simulink library "ann"  (Simulink 3.00)
undefined symbols (not defined in the file): V0, W0
libraries: simulink3 x3, neural x1
(part 2 of 2)

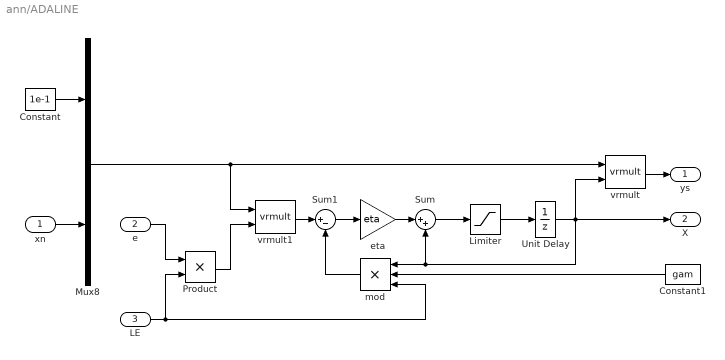
== system ann/ADALINE ==
  xn : Inport  Port=1  PortWidth=-1  SampleTime=-1  DataType=auto
      settings: SignalType=auto
  e : Inport  Port=2  PortWidth=-1  SampleTime=-1  DataType=auto
      settings: SignalType=auto
  LE : Inport  Port=3  PortWidth=-1  SampleTime=-1  DataType=auto
      settings: SignalType=auto
  Constant : Constant  Value=1e-1
  Constant1 : Constant  Orientation=left  Value=gam
  Limiter : Saturate  UpperLimit=L  LowerLimit=-L
  Mux8 : Mux  Inputs=2
  Product : Product  Inputs=2  SaturateOnIntegerOverflow=on
  Sum : Sum  Inputs=|++  SaturateOnIntegerOverflow=on
  Sum1 : Sum  Inputs=|+-  SaturateOnIntegerOverflow=on
  Unit Delay : UnitDelay  X0=W(:)  SampleTime=T
  eta : Gain  Gain=eta  SaturateOnIntegerOverflow=on
  mod : Product  Orientation=left  Inputs=3  SaturateOnIntegerOverflow=on
  vrmult : S-Function  FunctionName=vrmult  Parameters=dims  PortCounts=[]  SFunctionModules=''  mask(Simulink Matrix Library Block){dims=[1 ni+1 no]}
      mask prompts: dims "[n p m]"
      mask help:
      | Real Varying Matrices Multiplication
      |   Input 1   : elements of matrix X (n by p)
      |   Input 2   : elements of matrix Y (p by m)
      |   Output   : elements of matrix X*Y (n by m)
      mask Help:
      | <p>
      | Elements of input and output matrices are taken columnwise.
      | </p>
      | <p>
      | To use this block you should have the smxl library in your path.
      | </p>
      mask Display: disp('Z=X*Y')
  vrmult1 : S-Function  FunctionName=vrmult  Parameters=dims  PortCounts=[]  SFunctionModules=''  mask(Simulink Matrix Library Block){dims=[ni+1 1 no]}
      mask prompts: dims "[n p m]"
      mask help:
      | Real Varying Matrices Multiplication
      |   Input 1   : elements of matrix X (n by p)
      |   Input 2   : elements of matrix Y (p by m)
      |   Output   : elements of matrix X*Y (n by m)
      mask Help:
      | <p>
      | Elements of input and output matrices are taken columnwise.
      | </p>
      | <p>
      | To use this block you should have the smxl library in your path.
      | </p>
      mask Display: disp('Z=X*Y')
  ys : Outport  Port=1
  X : Outport  Port=2
  wires:
  Limiter/1 -> Unit Delay/1
  Sum/1 -> Limiter/1
  Unit Delay/1 -> vrmult/2, Sum/2, mod/1, X/1
  vrmult/1 -> ys/1
  Constant1/1 -> mod/2
  eta/1 -> Sum/1
  Sum1/1 -> eta/1
  vrmult1/1 -> Sum1/1
  mod/1 -> Sum1/2
  Product/1 -> vrmult1/2
  e/1 -> Product/1
  LE/1 -> Product/2, mod/3
  Mux8/1 -> vrmult/1, vrmult1/1
  xn/1 -> Mux8/2
  Constant/1 -> Mux8/1

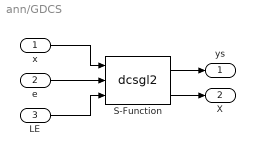
== system ann/GDCS ==
  x : Inport  Port=1  PortWidth=-1  SampleTime=-1  DataType=auto
      settings: SignalType=auto
  e : Inport  Port=2  PortWidth=-1  SampleTime=-1  DataType=auto
      settings: SignalType=auto
  LE : Inport  Port=3  PortWidth=-1  SampleTime=-1  DataType=auto
      settings: SignalType=auto
  S-Function : S-Function  FunctionName=dcsgl2  Parameters=Dim,norlat,eta,lim,real(lga),S,T  PortCounts=[]  SFunctionModules=''
  ys : Outport  Port=1
  X : Outport  Port=2
  wires:
  S-Function/1 -> ys/1
  S-Function/2 -> X/1
  x/1 -> S-Function/1
  e/1 -> S-Function/2
  LE/1 -> S-Function/3

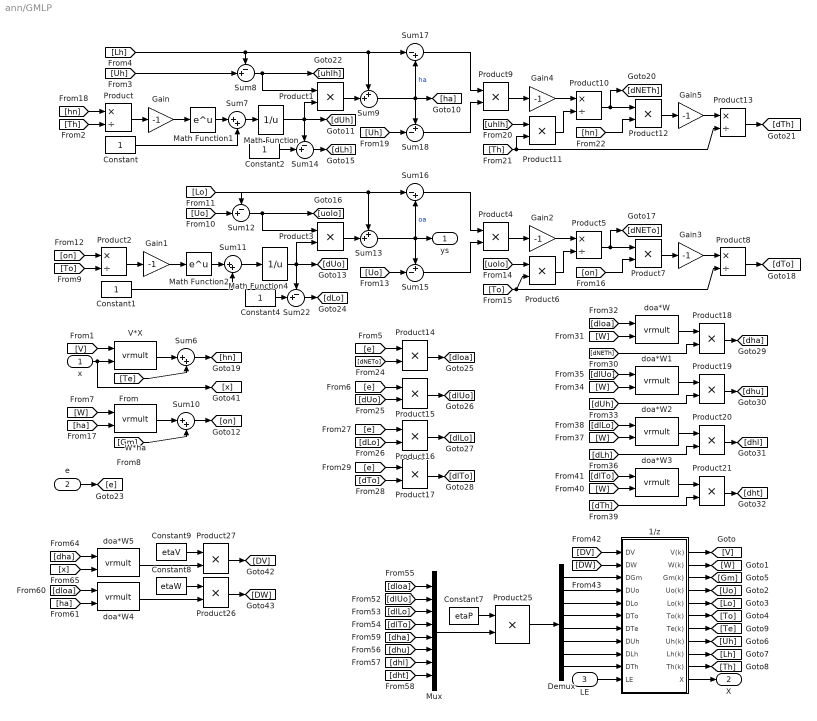
== system ann/GMLP ==
  x : Inport  Port=1  PortWidth=-1  SampleTime=-1  DataType=auto
      settings: SignalType=auto
  e : Inport  Port=2  PortWidth=-1  SampleTime=-1  DataType=auto
      settings: SignalType=auto
  LE : Inport  Port=3  PortWidth=-1  SampleTime=-1  DataType=auto
      settings: SignalType=auto
  1/z : Subsystem
  Constant{,1..2,4} (4 alike) : Constant  Value=1
  Constant7 : Constant  Value=etaP
  Constant8 : Constant  Value=etaW
  Constant9 : Constant  Value=etaV
  Demux : Demux  Outputs=8
  Gain{,1..5} (6 alike) : Gain  Gain=-1  SaturateOnIntegerOverflow=on
  Math Function : Math  Operator=reciprocal  OutputSignalType=auto
  Math Function1 : Math  Operator=exp  OutputSignalType=auto
  Math Function2 : Math  Operator=exp  OutputSignalType=auto
  Math Function4 : Math  Operator=reciprocal  OutputSignalType=auto
  Mux : Mux  Inputs=8
  Product{,2,5,8,10,13} (6 alike) : Product  Inputs=*/  SaturateOnIntegerOverflow=on
  Product{1,3..4,6..7,9,11..12,14..21,25..27} (19 alike) : Product  Inputs=**  SaturateOnIntegerOverflow=on
  Sum{6..7,10..11} (4 alike) : Sum  Inputs=|++  SaturateOnIntegerOverflow=on
  Sum{8,12,14,22} (4 alike) : Sum  Inputs=-+|  SaturateOnIntegerOverflow=on
  Sum13 : Sum  Inputs=++|  SaturateOnIntegerOverflow=on
  Sum15 : Sum  Inputs=+-|  SaturateOnIntegerOverflow=on
  Sum16 : Sum  Inputs=|-+  SaturateOnIntegerOverflow=on
  Sum17 : Sum  Inputs=|-+  SaturateOnIntegerOverflow=on
  Sum18 : Sum  Inputs=+-|  SaturateOnIntegerOverflow=on
  Sum9 : Sum  Inputs=++|  SaturateOnIntegerOverflow=on
  V*X : S-Function  FunctionName=vrmult  Parameters=dims  PortCounts=[]  SFunctionModules=''  mask(Simulink Matrix Library Block){dims=[nh ni 1]}
      mask prompts: dims "[n p m]"
      mask help:
      | Real Varying Matrices Multiplication
      |   Input 1   : elements of matrix X (n by p)
      |   Input 2   : elements of matrix Y (p by m)
      |   Output   : elements of matrix X*Y (n by m)
      mask Help:
      | <p>
      | Elements of input and output matrices are taken columnwise.
      | </p>
      | <p>
      | To use this block you should have the smxl library in your path.
      | </p>
      mask Display: disp('Z=X*Y')
  W*ha : S-Function  FunctionName=vrmult  Parameters=dims  PortCounts=[]  SFunctionModules=''  mask(Simulink Matrix Library Block){dims=[no nh 1]}
      mask prompts: dims "[n p m]"
      mask help:
      | Real Varying Matrices Multiplication
      |   Input 1   : elements of matrix X (n by p)
      |   Input 2   : elements of matrix Y (p by m)
      |   Output   : elements of matrix X*Y (n by m)
      mask Help:
      | <p>
      | Elements of input and output matrices are taken columnwise.
      | </p>
      | <p>
      | To use this block you should have the smxl library in your path.
      | </p>
      mask Display: disp('Z=X*Y')
  doa*W : S-Function  FunctionName=vrmult  Parameters=dims  PortCounts=[]  SFunctionModules=''  mask(Simulink Matrix Library Block){dims=[1 no nh]}
      mask prompts: dims "[n p m]"
      mask help:
      | Real Varying Matrices Multiplication
      |   Input 1   : elements of matrix X (n by p)
      |   Input 2   : elements of matrix Y (p by m)
      |   Output   : elements of matrix X*Y (n by m)
      mask Help:
      | <p>
      | Elements of input and output matrices are taken columnwise.
      | </p>
      | <p>
      | To use this block you should have the smxl library in your path.
      | </p>
      mask Display: disp('Z=X*Y')
  doa*W1 : S-Function  FunctionName=vrmult  Parameters=dims  PortCounts=[]  SFunctionModules=''  mask(Simulink Matrix Library Block){dims=[1 no nh]}
      mask prompts: dims "[n p m]"
      mask help:
      | Real Varying Matrices Multiplication
      |   Input 1   : elements of matrix X (n by p)
      |   Input 2   : elements of matrix Y (p by m)
      |   Output   : elements of matrix X*Y (n by m)
      mask Help:
      | <p>
      | Elements of input and output matrices are taken columnwise.
      | </p>
      | <p>
      | To use this block you should have the smxl library in your path.
      | </p>
      mask Display: disp('Z=X*Y')
  doa*W2 : S-Function  FunctionName=vrmult  Parameters=dims  PortCounts=[]  SFunctionModules=''  mask(Simulink Matrix Library Block){dims=[1 no nh]}
      mask prompts: dims "[n p m]"
      mask help:
      | Real Varying Matrices Multiplication
      |   Input 1   : elements of matrix X (n by p)
      |   Input 2   : elements of matrix Y (p by m)
      |   Output   : elements of matrix X*Y (n by m)
      mask Help:
      | <p>
      | Elements of input and output matrices are taken columnwise.
      | </p>
      | <p>
      | To use this block you should have the smxl library in your path.
      | </p>
      mask Display: disp('Z=X*Y')
  doa*W3 : S-Function  FunctionName=vrmult  Parameters=dims  PortCounts=[]  SFunctionModules=''  mask(Simulink Matrix Library Block){dims=[1 no nh]}
      mask prompts: dims "[n p m]"
      mask help:
      | Real Varying Matrices Multiplication
      |   Input 1   : elements of matrix X (n by p)
      |   Input 2   : elements of matrix Y (p by m)
      |   Output   : elements of matrix X*Y (n by m)
      mask Help:
      | <p>
      | Elements of input and output matrices are taken columnwise.
      | </p>
      | <p>
      | To use this block you should have the smxl library in your path.
      | </p>
      mask Display: disp('Z=X*Y')
  doa*W4 : S-Function  FunctionName=vrmult  Parameters=dims  PortCounts=[]  SFunctionModules=''  mask(Simulink Matrix Library Block){dims=[no 1 nh]}
      mask prompts: dims "[n p m]"
      mask help:
      | Real Varying Matrices Multiplication
      |   Input 1   : elements of matrix X (n by p)
      |   Input 2   : elements of matrix Y (p by m)
      |   Output   : elements of matrix X*Y (n by m)
      mask Help:
      | <p>
      | Elements of input and output matrices are taken columnwise.
      | </p>
      | <p>
      | To use this block you should have the smxl library in your path.
      | </p>
      mask Display: disp('Z=X*Y')
  doa*W5 : S-Function  FunctionName=vrmult  Parameters=dims  PortCounts=[]  SFunctionModules=''  mask(Simulink Matrix Library Block){dims=[nh 1 ni]}
      mask prompts: dims "[n p m]"
      mask help:
      | Real Varying Matrices Multiplication
      |   Input 1   : elements of matrix X (n by p)
      |   Input 2   : elements of matrix Y (p by m)
      |   Output   : elements of matrix X*Y (n by m)
      mask Help:
      | <p>
      | Elements of input and output matrices are taken columnwise.
      | </p>
      | <p>
      | To use this block you should have the smxl library in your path.
      | </p>
      mask Display: disp('Z=X*Y')
  ys : Outport  Port=1
  X : Outport  Port=2
  wires:
  Sum10/1 -> [on]
  1/z/11(X) -> X/1
  Product25/1 -> Demux/1
  Math Function2/1 -> Sum11/1
  Gain1/1 -> Math Function2/1
  1/z/10(Th(k)) -> [Th]
  1/z/9(Lh(k)) -> [Lh]
  1/z/8(Uh(k)) -> [Uh]
  1/z/7(Te(k)) -> [Te]
  1/z/6(To(k)) -> [To]
  1/z/5(Lo(k)) -> [Lo]
  1/z/4(Uo(k)) -> [Uo]
  1/z/3(Gm(k)) -> [Gm]
  1/z/2(W(k)) -> [W]
  1/z/1(V(k)) -> [V]
  [DV] -> 1/z/1(DV)
  [DW] -> 1/z/2(DW)
  Product27/1 -> [DV]
  Product26/1 -> [DW]
  doa*W4/1 -> Product26/2
  Constant8/1 -> Product26/1
  [dloa] -> doa*W4/1
  doa*W5/1 -> Product27/2
  Constant9/1 -> Product27/1
  [x] -> doa*W5/2
  [dha] -> doa*W5/1
  [ha] -> doa*W4/2
  Product18/1 -> [dha]
  Product17/1 -> [dlTo]
  [e] -> Product17/1
  Product16/1 -> [dlLo]
  [dLo] -> Product16/2
  [e] -> Product16/1
  Product15/1 -> [dlUo]
  [dUo] -> Product15/2
  [e] -> Product15/1
  Product14/1 -> [dloa]
  [dNETo] -> Product14/2
  [e] -> Product14/1
  x/1 -> [x], V*X/2
  Sum6/1 -> [hn]
  [V] -> V*X/1
  [Te] -> Sum6/2
  V*X/1 -> Sum6/1
  [ha] -> W*ha/2
  W*ha/1 -> Sum10/1
  [W] -> W*ha/1
  [Gm] -> Sum10/2
  [dTh] -> Product21/2
  Product21/1 -> [dht]
  doa*W3/1 -> Product21/1
  [W] -> doa*W3/2
  [dlTo] -> doa*W3/1
  [dLh] -> Product20/2
  Product20/1 -> [dhl]
  doa*W2/1 -> Product20/1
  [W] -> doa*W2/2
  [dlLo] -> doa*W2/1
  [dUh] -> Product19/2
  Product19/1 -> [dhu]
  doa*W1/1 -> Product19/1
  [W] -> doa*W1/2
  [dlUo] -> doa*W1/1
  [dNETh] -> Product18/2
  doa*W/1 -> Product18/1
  [W] -> doa*W/2
  [dloa] -> doa*W/1
  [dTo] -> Product17/2
  Sum22/1 -> [dLo]
  Constant4/1 -> Sum22/2
  Sum11/1 -> Math Function4/1
  [Lo] -> Sum16/1, Sum13/1, Sum12/1
  [Uo] -> Sum12/2
  Math Function4/1 -> Sum22/1, [dUo], Product3/2
  [on] -> Product2/1
  Constant1/1 -> Sum11/2
  Product2/1 -> Gain1/1
  [To] -> Product2/2
  Sum13/1 -> ys/1, Sum15/1, Sum16/2  "oa"
  Product3/1 -> Sum13/2
  [To] -> Product8/2, Product6/2
  Gain3/1 -> Product8/1
  Product7/1 -> Gain3/1
  Product5/1 -> Product7/1, [dNETo]
  Product6/1 -> Product5/2
  [uolo] -> Product6/1
  Gain2/1 -> Product5/1
  Sum12/1 -> [uolo], Product3/1
  Product4/1 -> Gain2/1
  Sum15/1 -> Product4/2
  Sum16/1 -> Product4/1
  [Uo] -> Sum15/2
  Product8/1 -> [dTo]
  Sum17/1 -> Product9/1
  Sum8/1 -> [uhlh], Product1/1
  [Lh] -> Sum17/1, Sum9/1, Sum8/1
  [Uh] -> Sum8/2
  Sum9/1 -> Sum18/1, [ha], Sum17/2  "ha"
  Product1/1 -> Sum9/2
  [Th] -> Product11/2, Product13/2
  Gain5/1 -> Product13/1
  Product12/1 -> Gain5/1
  [hn] -> Product12/2
  Product10/1 -> [dNETh], Product12/1
  Product11/1 -> Product10/2
  [uhlh] -> Product11/1
  Gain4/1 -> Product10/1
  Product9/1 -> Gain4/1
  Sum18/1 -> Product9/2
  Product13/1 -> [dTh]
  [Uh] -> Sum18/2
  [hn] -> Product/1
  Constant2/1 -> Sum14/2
  Sum14/1 -> [dLh]
  Math Function/1 -> Product1/2, Sum14/1, [dUh]
  Sum7/1 -> Math Function/1
  Constant/1 -> Sum7/2
  Math Function1/1 -> Sum7/1
  Gain/1 -> Math Function1/1
  Product/1 -> Gain/1
  [Th] -> Product/2
  Demux/1 -> 1/z/3(DGm)
  Demux/8 -> 1/z/10(DTh)
  Demux/7 -> 1/z/9(DLh)
  Demux/6 -> 1/z/8(DUh)
  Demux/5 -> 1/z/7(DTe)
  Demux/4 -> 1/z/6(DTo)
  Demux/3 -> 1/z/5(DLo)
  Demux/2 -> 1/z/4(DUo)
  e/1 -> [e]
  LE/1 -> 1/z/11(LE)
  Constant7/1 -> Product25/1
  [dht] -> Mux/8
  [dhl] -> Mux/7
  [dhu] -> Mux/6
  [dha] -> Mux/5
  [dlTo] -> Mux/4
  [dlLo] -> Mux/3
  [dloa] -> Mux/1
  [dlUo] -> Mux/2
  Mux/1 -> Product25/2
  [on] -> Product7/2

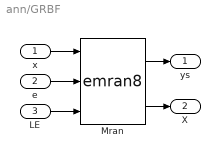
== system ann/GRBF ==
  x : Inport  Port=1  PortWidth=-1  SampleTime=-1  DataType=auto
      settings: SignalType=auto
  e : Inport  Port=2  PortWidth=-1  SampleTime=-1  DataType=auto
      settings: SignalType=auto
  LE : Inport  Port=3  PortWidth=-1  SampleTime=-1  DataType=auto
      settings: SignalType=auto
  Mran : S-Function  FunctionName=emran8  Parameters=real(dim(:)),real(nwrap(:)),real(eta(:)),real(gam(:)),real(lim(:)),real(e1(:)),real(e2(:)),real(e3(:)),real(x0(:)),real(T(:))  PortCounts=[]  SFunctionModules=''
  ys : Outport  Port=1
  X : Outport  Port=2
  wires:
  Mran/1 -> ys/1
  Mran/2 -> X/1
  x/1 -> Mran/1
  e/1 -> Mran/2
  LE/1 -> Mran/3

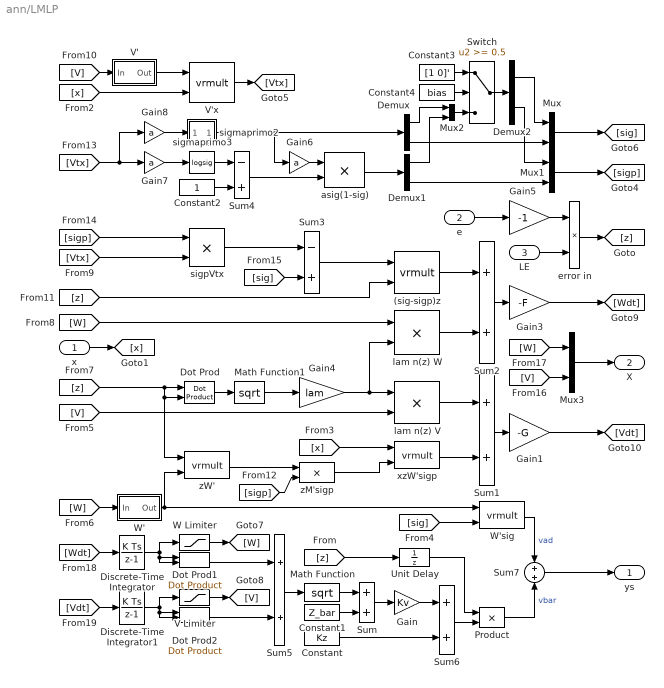
== system ann/LMLP ==
  x : Inport  Port=1  PortWidth=-1  SampleTime=-1  DataType=auto
      settings: SignalType=auto
  e : Inport  Port=2  PortWidth=-1  SampleTime=-1  DataType=auto
      settings: SignalType=auto
  LE : Inport  Port=3  PortWidth=-1  SampleTime=-1  DataType=auto
      settings: SignalType=auto
  (sig-sigp)z : S-Function  FunctionName=vrmult  Parameters=dims  PortCounts=[]  SFunctionModules=''  mask(Simulink Matrix Library Block){dims=[nnh 1 nno]}
      mask prompts: dims "[n p m]"
      mask help:
      | Real Varying Matrices Multiplication
      |   Input 1   : elements of matrix X (n by p)
      |   Input 2   : elements of matrix Y (p by m)
      |   Output   : elements of matrix X*Y (n by m)
      mask Help:
      | <p>
      | Elements of input and output matrices are taken columnwise.
      | </p>
      | <p>
      | To use this block you should have the smxl library in your path.
      | </p>
      mask Display: disp('Z=X*Y')
  Constant : Constant  Value=Kz
  Constant1 : Constant  Value=Z_bar
  Constant2 : Constant  Value=1
  Constant3 : Constant  Value=[1 0]'
  Constant4 : Constant  Value=bias
  Demux : Demux  Outputs=[1 nnh-1]
  Demux1 : Demux  Outputs=[1 nnh-1]
  Demux2 : Demux  Outputs=[1 1]
  Discrete-Time Integrator : DiscreteIntegrator  IntegratorMethod=ForwardEuler  ExternalReset=none  InitialConditionSource=internal  InitialCondition=W0(:)  LimitOutput=off  UpperSaturationLimit=inf  LowerSaturationLimit=-inf  ShowSaturationPort=off  ShowStatePort=off  SampleTime=T
  Discrete-Time Integrator1 : DiscreteIntegrator  IntegratorMethod=ForwardEuler  ExternalReset=none  InitialConditionSource=internal  InitialCondition=V0(:)  LimitOutput=off  UpperSaturationLimit=inf  LowerSaturationLimit=-inf  ShowSaturationPort=off  ShowStatePort=off  SampleTime=T
  Dot Prod : simulink3/Math/Dot Product
  Dot Prod1 : simulink3/Math/Dot Product
  Dot Prod2 : simulink3/Math/Dot Product
  Gain : Gain  Gain=Kv  SaturateOnIntegerOverflow=on
  Gain1 : Gain  Gain=-G  SaturateOnIntegerOverflow=on
  Gain3 : Gain  Gain=-F  SaturateOnIntegerOverflow=on
  Gain4 : Gain  Gain=lam  SaturateOnIntegerOverflow=on
  Gain5 : Gain  Gain=-1  SaturateOnIntegerOverflow=on
  Gain6 : Gain  Gain=a  SaturateOnIntegerOverflow=on
  Gain7 : Gain  Gain=a  SaturateOnIntegerOverflow=on
  Gain8 : Gain  Gain=a  SaturateOnIntegerOverflow=on
  Math Function : Math  Operator=sqrt  OutputSignalType=real
  Math Function1 : Math  Operator=sqrt  OutputSignalType=real
  Mux : Mux  Inputs=[1 nnh-1]
  Mux1 : Mux  Inputs=[1 nnh-1]
  Mux2 : Mux  Inputs=[1 1]
  Mux3 : Mux  Inputs=2
  Product : Product  Inputs=2  SaturateOnIntegerOverflow=on
  Sum{,1..2,5..6} (5 alike) : Sum  Inputs=++  SaturateOnIntegerOverflow=on
  Sum3 : Sum  Inputs=-+  SaturateOnIntegerOverflow=on
  Sum4 : Sum  Inputs=-+  SaturateOnIntegerOverflow=on
  Sum7 : Sum  Inputs=+|+  SaturateOnIntegerOverflow=on
  Switch : Switch  Threshold=0.5
  Unit Delay : UnitDelay  X0=0  SampleTime=T
  V Limiter : Saturate  UpperLimit=LV  LowerLimit=-LV
  V' : Subsystem  mask(Simulink Matrix Library Block){dims=[nni nnh]}
      mask prompts: dims "[n m]"
      mask help:
      | Real Varying Matrix Transposition
      |   Input      : elements of matrix X (n by m)
      |   Output   : elements of matrix X' (m by n)
      mask Help:
      | <p>
      | Elements of input and output matrices are taken columnwise.
      | </p>
      | <p>
      | To use this block you should have the smxl library in your path.
      | </p>
      mask Display: disp('Y=X''')
  V'x : S-Function  FunctionName=vrmult  Parameters=dims  PortCounts=[]  SFunctionModules=''  mask(Simulink Matrix Library Block){dims=[nnh nni 1]}
      mask prompts: dims "[n p m]"
      mask help:
      | Real Varying Matrices Multiplication
      |   Input 1   : elements of matrix X (n by p)
      |   Input 2   : elements of matrix Y (p by m)
      |   Output   : elements of matrix X*Y (n by m)
      mask Help:
      | <p>
      | Elements of input and output matrices are taken columnwise.
      | </p>
      | <p>
      | To use this block you should have the smxl library in your path.
      | </p>
      mask Display: disp('Z=X*Y')
  W Limiter : Saturate  UpperLimit=LW  LowerLimit=-LW
  W' : Subsystem  mask(Simulink Matrix Library Block){dims=[nnh nno]}
      mask prompts: dims "[n m]"
      mask help:
      | Real Varying Matrix Transposition
      |   Input      : elements of matrix X (n by m)
      |   Output   : elements of matrix X' (m by n)
      mask Help:
      | <p>
      | Elements of input and output matrices are taken columnwise.
      | </p>
      | <p>
      | To use this block you should have the smxl library in your path.
      | </p>
      mask Display: disp('Y=X''')
  W'sig : S-Function  FunctionName=vrmult  Parameters=dims  PortCounts=[]  SFunctionModules=''  mask(Simulink Matrix Library Block){dims=[nno nnh 1]}
      mask prompts: dims "[n p m]"
      mask help:
      | Real Varying Matrices Multiplication
      |   Input 1   : elements of matrix X (n by p)
      |   Input 2   : elements of matrix Y (p by m)
      |   Output   : elements of matrix X*Y (n by m)
      mask Help:
      | <p>
      | Elements of input and output matrices are taken columnwise.
      | </p>
      | <p>
      | To use this block you should have the smxl library in your path.
      | </p>
      mask Display: disp('Z=X*Y')
  asig(1-sig) : Product  Inputs=2  SaturateOnIntegerOverflow=on
  error in : Product  Inputs=2  SaturateOnIntegerOverflow=on
  lam n(z) V : Product  Inputs=2  SaturateOnIntegerOverflow=on
  lam n(z) W : Product  Inputs=2  SaturateOnIntegerOverflow=on
  sigmaprimo2 : Subsystem
      mask Description: Log sigmoid transfer function
      mask Display: plot([-1 1],[0 0],[-1 -.9 -.8 -.7 -.6 -.5 -.4 -.3 -.2 -.1 0 .1 .2 .3 .4 .5 .6 .7 .8 .9 1],1./(1+exp(-8*[-1 -.9 -.8 -.7 -.6 -.5 -.4 -.3 -.2 -.1 0 .1 .2 .3 .4 .5 .6 .7 .8 .9 1]))+.01)
  sigmaprimo3 : neural/Transfer Functions/logsig
  sigpVtx : Product  Inputs=2  SaturateOnIntegerOverflow=on
  xzW'sigp : S-Function  FunctionName=vrmult  Parameters=dims  PortCounts=[]  SFunctionModules=''  mask(Simulink Matrix Library Block){dims=[nni 1 nnh]}
      mask prompts: dims "[n p m]"
      mask help:
      | Real Varying Matrices Multiplication
      |   Input 1   : elements of matrix X (n by p)
      |   Input 2   : elements of matrix Y (p by m)
      |   Output   : elements of matrix X*Y (n by m)
      mask Help:
      | <p>
      | Elements of input and output matrices are taken columnwise.
      | </p>
      | <p>
      | To use this block you should have the smxl library in your path.
      | </p>
      mask Display: disp('Z=X*Y')
  zM'sigp : Product  Inputs=2  SaturateOnIntegerOverflow=on
  zW' : S-Function  FunctionName=vrmult  Parameters=dims  PortCounts=[]  SFunctionModules=''  mask(Simulink Matrix Library Block){dims=[1 nno nnh]}
      mask prompts: dims "[n p m]"
      mask help:
      | Real Varying Matrices Multiplication
      |   Input 1   : elements of matrix X (n by p)
      |   Input 2   : elements of matrix Y (p by m)
      |   Output   : elements of matrix X*Y (n by m)
      mask Help:
      | <p>
      | Elements of input and output matrices are taken columnwise.
      | </p>
      | <p>
      | To use this block you should have the smxl library in your path.
      | </p>
      mask Display: disp('Z=X*Y')
  ys : Outport  Port=1
  X : Outport  Port=2
  wires:
  Gain5/1 -> error in/1
  e/1 -> Gain5/1
  Unit Delay/1 -> Product/1
  [z] -> Unit Delay/1
  [V] -> lam n(z) V/2
  x/1 -> [x]
  [V] -> V'/1(In)
  V'/1(Out) -> V'x/1
  [x] -> V'x/2
  V'x/1 -> [Vtx]
  Constant3/1 -> Switch/1
  Constant4/1 -> Switch/2
  Mux2/1 -> Switch/3
  Switch/1 -> Demux2/1
  Demux2/2 -> Mux1/1
  Demux2/1 -> Mux/1
  Demux/1 -> Mux2/1
  Demux1/1 -> Mux2/2
  error in/1 -> [z]
  LE/1 -> error in/2
  [W] -> Mux3/1
  [V] -> Mux3/2
  Mux3/1 -> X/1
  Constant1/1 -> Sum/2
  Math Function/1 -> Sum/1
  Sum/1 -> Gain/1
  Gain/1 -> Sum6/1
  Constant/1 -> Sum6/2
  Sum6/1 -> Product/2
  [sig] -> W'sig/2
  W'sig/1 -> Sum7/1  "vad"
  Product/1 -> Sum7/2  "vbar"
  Sum5/1 -> Math Function/1
  V Limiter/1 -> [V]
  W Limiter/1 -> [W]
  [Vdt] -> Discrete-Time Integrator1/1
  [Wdt] -> Discrete-Time Integrator/1
  Dot Prod2/1 -> Sum5/2
  Dot Prod1/1 -> Sum5/1
  [W] -> W'/1(In)
  Sum7/1 -> ys/1
  Gain1/1 -> [Vdt]
  Sum2/1 -> Gain3/1
  (sig-sigp)z/1 -> Sum2/1
  lam n(z) W/1 -> Sum2/2
  Gain4/1 -> lam n(z) V/1, lam n(z) W/2
  [z] -> Dot Prod/1, zW'/1, Dot Prod/2
  [W] -> lam n(z) W/1
  [sigp] -> sigpVtx/1
  [Vtx] -> sigpVtx/2
  Sum3/1 -> (sig-sigp)z/1
  [sig] -> Sum3/2
  sigpVtx/1 -> Sum3/1
  [z] -> (sig-sigp)z/2
  Dot Prod/1 -> Math Function1/1
  Math Function1/1 -> Gain4/1
  Sum1/1 -> Gain1/1
  lam n(z) V/1 -> Sum1/1
  xzW'sigp/1 -> Sum1/2
  [x] -> xzW'sigp/1
  zM'sigp/1 -> xzW'sigp/2
  zW'/1 -> zM'sigp/1
  [sigp] -> zM'sigp/2
  W'/1(Out) -> zW'/2, W'sig/1
  Gain3/1 -> [Wdt]
  Mux/1 -> [sig]
  Mux1/1 -> [sigp]
  Demux/2 -> Mux/2
  Demux1/2 -> Mux1/2
  Gain6/1 -> asig(1-sig)/1
  asig(1-sig)/1 -> Demux1/1
  Constant2/1 -> Sum4/2
  Gain7/1 -> sigmaprimo3/1
  Gain8/1 -> sigmaprimo2/1(n)
  [Vtx] -> Gain7/1, Gain8/1
  sigmaprimo3/1 -> Sum4/1
  Sum4/1 -> asig(1-sig)/2
  sigmaprimo2/1(a) -> Gain6/1, Demux/1
  Discrete-Time Integrator/1 -> W Limiter/1, Dot Prod1/1, Dot Prod1/2
  Discrete-Time Integrator1/1 -> V Limiter/1, Dot Prod2/1, Dot Prod2/2

== system ann/Pid Demo F4 ==

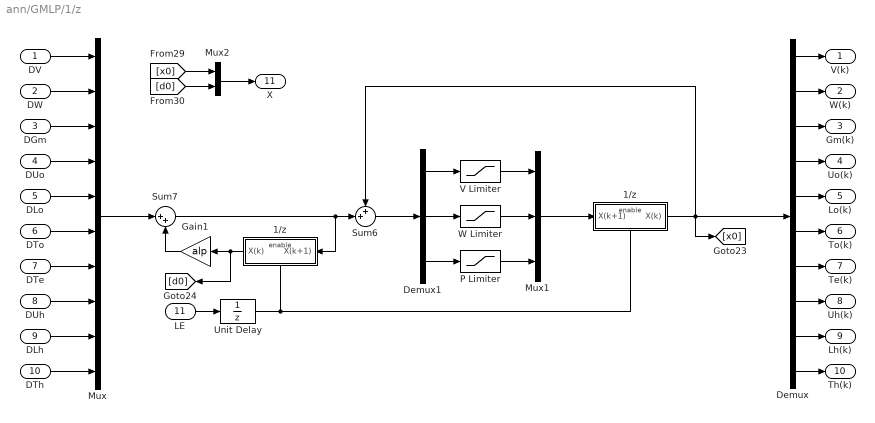
== system ann/GMLP/1/z ==
  DV : Inport  Port=1  PortWidth=-1  SampleTime=-1  DataType=auto
      settings: SignalType=auto
  DW : Inport  Port=2  PortWidth=-1  SampleTime=-1  DataType=auto
      settings: SignalType=auto
  DGm : Inport  Port=3  PortWidth=-1  SampleTime=-1  DataType=auto
      settings: SignalType=auto
  DUo : Inport  Port=4  PortWidth=-1  SampleTime=-1  DataType=auto
      settings: SignalType=auto
  DLo : Inport  Port=5  PortWidth=-1  SampleTime=-1  DataType=auto
      settings: SignalType=auto
  DTo : Inport  Port=6  PortWidth=-1  SampleTime=-1  DataType=auto
      settings: SignalType=auto
  DTe : Inport  Port=7  PortWidth=-1  SampleTime=-1  DataType=auto
      settings: SignalType=auto
  DUh : Inport  Port=8  PortWidth=-1  SampleTime=-1  DataType=auto
      settings: SignalType=auto
  DLh : Inport  Port=9  PortWidth=-1  SampleTime=-1  DataType=auto
      settings: SignalType=auto
  DTh : Inport  Port=10  PortWidth=-1  SampleTime=-1  DataType=auto
      settings: SignalType=auto
  LE : Inport  Port=11  PortWidth=-1  SampleTime=-1  DataType=auto
      settings: SignalType=auto
  1/z : Subsystem  Orientation=left
  "1/z " : Subsystem
  Demux : Demux  Outputs=[nh*ni no*nh no no no no nh nh nh nh]
  Demux1 : Demux  Outputs=[nh*ni no*nh 4*(no+nh)]
  Gain1 : Gain  Orientation=left  Gain=alp  SaturateOnIntegerOverflow=on
  Mux : Mux  Inputs=[nh*ni no*nh no no no no nh nh nh nh]
  Mux1 : Mux  Inputs=[nh*ni no*nh 4*(no+nh)]
  Mux2 : Mux  Inputs=2
  P Limiter : Saturate  UpperLimit=L(3)  LowerLimit=-L(3)
  Sum6 : Sum  Inputs=++|  SaturateOnIntegerOverflow=on
  Sum7 : Sum  Inputs=|++  SaturateOnIntegerOverflow=on
  Unit Delay : UnitDelay  X0=1  SampleTime=T
  V Limiter : Saturate  UpperLimit=L(1)  LowerLimit=-L(1)
  W Limiter : Saturate  UpperLimit=L(2)  LowerLimit=-L(2)
  V(k) : Outport  Port=1
  W(k) : Outport  Port=2
  Gm(k) : Outport  Port=3
  Uo(k) : Outport  Port=4
  Lo(k) : Outport  Port=5
  To(k) : Outport  Port=6
  Te(k) : Outport  Port=7
  Uh(k) : Outport  Port=8
  Lh(k) : Outport  Port=9
  Th(k) : Outport  Port=10
  X : Outport  Port=11
  wires:
  P Limiter/1 -> Mux1/3
  Demux1/3 -> P Limiter/1
  W Limiter/1 -> Mux1/2
  Demux1/2 -> W Limiter/1
  V Limiter/1 -> Mux1/1
  Demux1/1 -> V Limiter/1
  Mux1/1 -> "1/z "/1(X(k+1))
  "1/z "/1(X(k)) -> Demux/1, Sum6/1, [x0]
  Demux/10 -> Th(k)/1
  Demux/9 -> Lh(k)/1
  Demux/8 -> Uh(k)/1
  Demux/7 -> Te(k)/1
  Demux/6 -> To(k)/1
  Demux/5 -> Lo(k)/1
  Demux/4 -> Uo(k)/1
  Demux/3 -> Gm(k)/1
  Demux/2 -> W(k)/1
  Demux/1 -> V(k)/1
  Mux2/1 -> X/1
  [d0] -> Mux2/2
  [x0] -> Mux2/1
  Sum6/1 -> Demux1/1
  DTh/1 -> Mux/10
  DLh/1 -> Mux/9
  DUh/1 -> Mux/8
  DTe/1 -> Mux/7
  DTo/1 -> Mux/6
  DLo/1 -> Mux/5
  DUo/1 -> Mux/4
  DGm/1 -> Mux/3
  DW/1 -> Mux/2
  DV/1 -> Mux/1
  Sum7/1 -> 1/z/1(X(k+1)), Sum6/2
  Gain1/1 -> Sum7/2
  Mux/1 -> Sum7/1
  1/z/1(X(k)) -> Gain1/1, [d0]
  Unit Delay/1 -> 1/z/Enable, "1/z "/Enable
  LE/1 -> Unit Delay/1

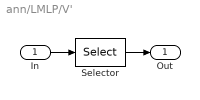
== system ann/LMLP/V' ==
  In : Inport  Port=1  PortWidth=-1  SampleTime=-1  DataType=auto
      settings: SignalType=auto
  Selector : Selector  Elements=reshape(reshape(1:dims(1)*dims(2),dims(1),dims(2))',dims(1)*dims(2),1)  InputPortWidth=dims(1)*dims(2)
  Out : Outport  Port=1
  wires:
  Selector/1 -> Out/1
  In/1 -> Selector/1

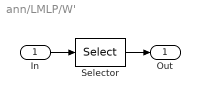
== system ann/LMLP/W' ==
  In : Inport  Port=1  PortWidth=-1  SampleTime=-1  DataType=auto
      settings: SignalType=auto
  Selector : Selector  Elements=reshape(reshape(1:dims(1)*dims(2),dims(1),dims(2))',dims(1)*dims(2),1)  InputPortWidth=dims(1)*dims(2)
  Out : Outport  Port=1
  wires:
  Selector/1 -> Out/1
  In/1 -> Selector/1

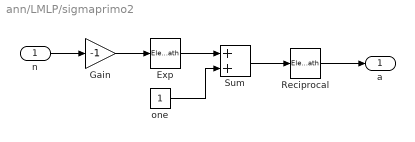
== system ann/LMLP/sigmaprimo2 ==
  n : Inport  Port=1  PortWidth=-1  SampleTime=-1  DataType=auto
      settings: SignalType=auto
  Exp : ElementaryMath  Operator=exp
  Gain : Gain  Gain=-1  SaturateOnIntegerOverflow=on
  Reciprocal : ElementaryMath  Operator=reciprocal
  Sum : Sum  Inputs=++  SaturateOnIntegerOverflow=on
  one : Constant  Value=1
  a : Outport  Port=1  InitialOutput=0
  wires:
  Reciprocal/1 -> a/1
  Sum/1 -> Reciprocal/1
  one/1 -> Sum/2
  Exp/1 -> Sum/1
  Gain/1 -> Exp/1
  n/1 -> Gain/1

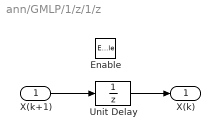
== system ann/GMLP/1/z/1/z ==
  X(k+1) : Inport  Port=1  PortWidth=-1  SampleTime=-1  DataType=auto
      settings: SignalType=auto
  Enable : EnablePort
  Unit Delay : UnitDelay  X0=d0  SampleTime=T
  X(k) : Outport  Port=1
  wires:
  Unit Delay/1 -> X(k)/1
  X(k+1)/1 -> Unit Delay/1

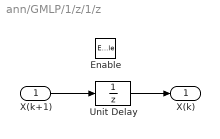
== system ann/GMLP/1/z/1/z  ==
  X(k+1) : Inport  Port=1  PortWidth=-1  SampleTime=-1  DataType=auto
      settings: SignalType=auto
  Enable : EnablePort
  Unit Delay : UnitDelay  X0=x0  SampleTime=T
  X(k) : Outport  Port=1
  wires:
  X(k+1)/1 -> Unit Delay/1
  Unit Delay/1 -> X(k)/1
